simulink model "practica2"  (Simulink 7.3)
settings: Solver=ode45  StartTime=0.0  StopTime=1000  RelTol=1e-3
undefined symbols (not defined in the file or in its folder): p
libraries: simeventsrouting1 x8, simeventssink1 x6, simeventsgenerators1 x4, simeventsattributes2 x4, simeventstiming1 x4, simeventsqueue1 x2, simeventsgates1 x2, simeventsserver1 x2
settings Model: Creator=Mario  LastModifiedBy=usuario
settings SimEventsCC: propDiagAttribOutput=1  propDiagFcnCallOutput=1  propDiagStatOutput=0

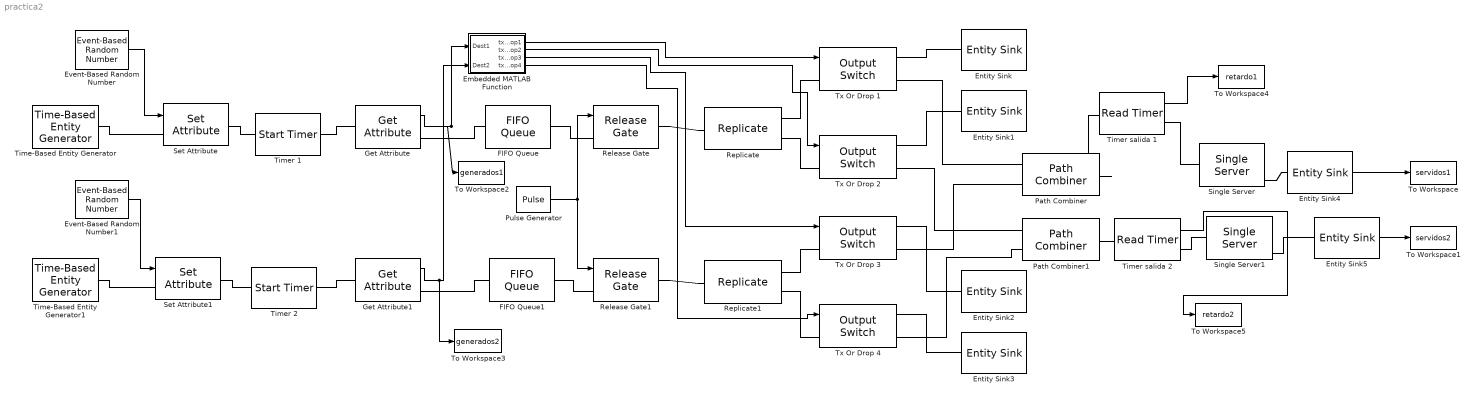
== system practica2 ==
  Embedded MATLAB Function : Stateflow chart
  Entity Sink{,1..3} (4 alike) : simeventssink1/Entity Sink  Priority=1  SystemSampleTime=-1  AvailableForArrivals=on  StatNumberArrived=Off
  Entity Sink4 : simeventssink1/Entity Sink  Priority=1  SystemSampleTime=-1  AvailableForArrivals=on  StatNumberArrived=On
  Entity Sink5 : simeventssink1/Entity Sink  Priority=1  SystemSampleTime=-1  AvailableForArrivals=on  StatNumberArrived=On
  Event-Based Random Number : simeventsgenerators1/Signal Generators/Event-Based Random Number  SystemSampleTime=-1  distribution=Arbitrary discrete  meanExp=1  minUnif=1  maxUnif=1  pOneBern=0.25  pSuccessBino=0.5  numTrialBino=1  meanNorm=0  stdNorm=1  minTri=1  maxTri=3  modeTri=2  thresholdLogn=0  scaleLogn=1  shapeLogn=1  pSuccessGeo=0.5  meanPoiss=1  thresholdLogl=0  scaleLogl=1  thresholdGam=0  scaleGam=1  shapeGam=1  minBeta=0  maxBeta=1  shape1Beta=1  shape2Beta=1  minUnid=0  maxUnid=1  numValueUnid=2  thresholdWbl=0  scaleWbl=1  shapeWbl=1  valueVecCont=[0 1]  cdfVecCont=[0 1]  valueVecDisc=[0 1 2]  probVecDisc=[1-p p/2 p/2]  seed=12345  IsProcessed=on  isConnected=1
  Event-Based Random Number1 : simeventsgenerators1/Signal Generators/Event-Based Random Number  SystemSampleTime=-1  distribution=Arbitrary discrete  meanExp=1  minUnif=1  maxUnif=1  pOneBern=0.25  pSuccessBino=0.5  numTrialBino=1  meanNorm=0  stdNorm=1  minTri=1  maxTri=3  modeTri=2  thresholdLogn=0  scaleLogn=1  shapeLogn=1  pSuccessGeo=0.5  meanPoiss=1  thresholdLogl=0  scaleLogl=1  thresholdGam=0  scaleGam=1  shapeGam=1  minBeta=0  maxBeta=1  shape1Beta=1  shape2Beta=1  minUnid=0  maxUnid=1  numValueUnid=2  thresholdWbl=0  scaleWbl=1  shapeWbl=1  valueVecCont=[0 1]  cdfVecCont=[0 1]  valueVecDisc=[0 1 2]  probVecDisc=[1-p p/2 p/2]  seed=76543  IsProcessed=on  isConnected=1
  FIFO Queue : simeventsqueue1/FIFO Queue  Priority=1  SystemSampleTime=-1  Capacity=1  EnableTOPort=off  StatNumberDeparted=Off  StatNumberInBlock=Off  StatPendingEntity=Off  StatAverageWait=Off  StatAverageQueueLength=Off  StatNumberTimedout=Off
  FIFO Queue1 : simeventsqueue1/FIFO Queue  Priority=1  SystemSampleTime=-1  Capacity=1  EnableTOPort=off  StatNumberDeparted=Off  StatNumberInBlock=Off  StatPendingEntity=Off  StatAverageWait=Off  StatAverageQueueLength=Off  StatNumberTimedout=Off
  Get Attribute : simeventsattributes2/Get Attribute  Priority=1  DialogController=des_ddg_create  DialogControllerArgs=DataTag9  SystemSampleTime=-1  AttributeName=Attribute1  AttributeMissing=Error  AttributeDefaultValue=1  AttributeSendTiming=After entity departure  AttributeTreatAsVector=1  StatNumberDeparted=Off  EvaluatedDefaultAttributeValue={[]}
  Get Attribute1 : simeventsattributes2/Get Attribute  Priority=1  DialogController=des_ddg_create  DialogControllerArgs=DataTag11  SystemSampleTime=-1  AttributeName=Attribute1  AttributeMissing=Error  AttributeDefaultValue=1  AttributeSendTiming=After entity departure  AttributeTreatAsVector=1  StatNumberDeparted=Off  EvaluatedDefaultAttributeValue={[]}
  Path Combiner : simeventsrouting1/Path Combiner  Priority=1  SystemSampleTime=-1  NumberInputPorts=2  InputPortPrecedence=IN1 port  InitialSeed=45675  SpecifyEventPriority=off  PriorityPathCombinerPortPrecedenceSelection=4100  StatNumberDeparted=Off  StatLastArrivalPort=Off  EvaluatedNumPorts=2
  Path Combiner1 : simeventsrouting1/Path Combiner  Priority=1  SystemSampleTime=-1  NumberInputPorts=2  InputPortPrecedence=IN1 port  InitialSeed=45675  SpecifyEventPriority=off  PriorityPathCombinerPortPrecedenceSelection=4100  StatNumberDeparted=Off  StatLastArrivalPort=Off  EvaluatedNumPorts=2
  Pulse Generator : DiscretePulseGenerator  Amplitude=1  Period=10  PulseWidth=5  PhaseDelay=3  SampleTime=0.1
  Release Gate : simeventsgates1/Release Gate  Priority=1  SystemSampleTime=-1  OpenGateUpon=Change in signal from port vc  SignalEdgeOption=Rising  SpecifyEventPriority=off  PriorityGateRelease=2200  StatNumberDeparted=Off
  Release Gate1 : simeventsgates1/Release Gate  Priority=1  SystemSampleTime=-1  OpenGateUpon=Change in signal from port vc  SignalEdgeOption=Rising  SpecifyEventPriority=off  PriorityGateRelease=2200  StatNumberDeparted=Off
  Replicate : simeventsrouting1/Replicate  Priority=1  SystemSampleTime=-1  NumberOutputPorts=2  ReplicateEntityWhen=All entity output ports are not blocked  OutputPortPrecedence=OUT1 port  InitialSeed=56789  ActionUponBlocking=Discard entity  StatNumberArrived=Off  StatNumberDeparted=Off  EvaluatedNumPorts=2
  Replicate1 : simeventsrouting1/Replicate  Priority=1  SystemSampleTime=-1  NumberOutputPorts=2  ReplicateEntityWhen=All entity output ports are not blocked  OutputPortPrecedence=OUT1 port  InitialSeed=56789  ActionUponBlocking=Discard entity  StatNumberArrived=Off  StatNumberDeparted=Off  EvaluatedNumPorts=2
  Set Attribute : simeventsattributes2/Set Attribute  Priority=1  DialogController=des_ddg_create  DialogControllerArgs=DataTag19  SystemSampleTime=-1  AttributeFrom=Signal port  AttributeName=Attribute1  AttributeTreatAsVector=1  AttributeValue=1  AttributeCreate=on  StatNumberDeparted=Off  EvaluatedAttributeValue={[]}
  Set Attribute1 : simeventsattributes2/Set Attribute  Priority=1  DialogController=des_ddg_create  DialogControllerArgs=DataTag21  SystemSampleTime=-1  AttributeFrom=Signal port  AttributeName=Attribute1  AttributeTreatAsVector=1  AttributeValue=1  AttributeCreate=on  StatNumberDeparted=Off  EvaluatedAttributeValue={[]}
  Single Server : simeventsserver1/Single Server  Priority=1  SystemSampleTime=-1  ServiceTimeFrom=Dialog  ServiceTime=0.99999  AttributeName=ServiceTime  PriorityServiceCompletion=500  PermitPreemption=off  SortingAttributeName=PriorityAttributeName  SortingDirection=Ascending  WriteToAttribute=off  ResidualAttributeName=ResidualServiceTime  CreateAttribute=on  EnableTOPort=off  StatNumberDeparted=On  StatNumberInBlock=Off  StatNumberPreempted=Off  StatPendingEntity=Off  StatAverageWait=Off  StatUtilization=On  StatNumberTimedout=Off
  Single Server1 : simeventsserver1/Single Server  Priority=1  SystemSampleTime=-1  ServiceTimeFrom=Dialog  ServiceTime=0.99999  AttributeName=ServiceTime  PriorityServiceCompletion=500  PermitPreemption=off  SortingAttributeName=PriorityAttributeName  SortingDirection=Ascending  WriteToAttribute=off  ResidualAttributeName=ResidualServiceTime  CreateAttribute=on  EnableTOPort=off  StatNumberDeparted=On  StatNumberInBlock=Off  StatNumberPreempted=Off  StatPendingEntity=Off  StatAverageWait=Off  StatUtilization=On  StatNumberTimedout=Off
  Time-Based Entity Generator : simeventsgenerators1/Entity Generators/Time-Based Entity Generator  Priority=1  DialogController=des_ddg_create  DialogControllerArgs=DataTag25  SystemSampleTime=-1  GenerateEntitiesUpon=Intergeneration time from dialog  Distribution=Constant  Minimum=0  Maximum=1  Mean=1  InitialSeed=12345  Period=1  PriorityEntityGeneration=300  GenerateEntityAtSimulationStart=on  ResponseWhenBlocked=Pause generation  ResponseWhenUnblocked=Immediate restart  EntityType=Blank  StatNumberDeparted=Off  StatPendingEntity=Off  StatAverageIntergenerationTime=Off
  Time-Based Entity Generator1 : simeventsgenerators1/Entity Generators/Time-Based Entity Generator  Priority=1  DialogController=des_ddg_create  DialogControllerArgs=DataTag27  SystemSampleTime=-1  GenerateEntitiesUpon=Intergeneration time from dialog  Distribution=Constant  Minimum=0  Maximum=1  Mean=1  InitialSeed=12345  Period=1  PriorityEntityGeneration=300  GenerateEntityAtSimulationStart=on  ResponseWhenBlocked=Pause generation  ResponseWhenUnblocked=Immediate restart  EntityType=Blank  StatNumberDeparted=Off  StatPendingEntity=Off  StatAverageIntergenerationTime=Off
  Timer 1 : simeventstiming1/Start Timer  Priority=0  SystemSampleTime=-1  TimerTag=T1  TimerStartedOption=Warn and continue  StatNumberDeparted=Off
  Timer 2 : simeventstiming1/Start Timer  Priority=0  SystemSampleTime=-1  TimerTag=T1  TimerStartedOption=Warn and continue  StatNumberDeparted=Off
  Timer salida 1 : simeventstiming1/Read Timer  Priority=0  SystemSampleTime=-1  TimerTag=T1  TimerModeOption=Error  TimerStop=off  StatNumberDeparted=Off  StatTimerNumberDeparted=Off  StatTimeElapsed=On  StatAverageTimeElapsed=Off
  Timer salida 2 : simeventstiming1/Read Timer  Priority=0  SystemSampleTime=-1  TimerTag=T1  TimerModeOption=Error  TimerStop=off  StatNumberDeparted=Off  StatTimerNumberDeparted=Off  StatTimeElapsed=On  StatAverageTimeElapsed=Off
  To Workspace : ToWorkspace  VariableName=servidos1  SampleTime=-1  SaveFormat=Array
  To Workspace1 : ToWorkspace  VariableName=servidos2  SampleTime=-1  SaveFormat=Array
  To Workspace2 : ToWorkspace  VariableName=generados1  SampleTime=1  SaveFormat=Array
  To Workspace3 : ToWorkspace  VariableName=generados2  SampleTime=1  SaveFormat=Array
  To Workspace4 : ToWorkspace  VariableName=retardo1  SampleTime=-1  SaveFormat=Array
  To Workspace5 : ToWorkspace  VariableName=retardo2  SampleTime=-1  SaveFormat=Array
  Tx Or Drop {1..4} (4 alike) : simeventsrouting1/Output Switch  Priority=1  SystemSampleTime=-1  NumberOutputPorts=2  SwitchingCriterion=From signal port p  InitialSeed=34567  AttributeName=Attribute1  InitialConditionsOpt=off  InitialConditions=1  EntityBufferOpt=off  SpecifyEventPriority=off  PriorityOutputSwitchSelectPort=4100  TimeoutPortOpt=off  StatNumberDeparted=Off  StatNumberTimedOut=Off  StatPendingEntity=Off  StatLastDeparturePort=Off  EvaluatedNumPorts=2
  wires:
  Event-Based Random Number/1 -> Set Attribute/1
  Event-Based Random Number1/1 -> Set Attribute1/1
  Get Attribute1/1 -> Embedded MATLAB Function/2(Dest2), To Workspace3/1
  Get Attribute/1 -> Embedded MATLAB Function/1(Dest1), To Workspace2/1
  Pulse Generator/1 -> Release Gate/1, Release Gate1/1
  Embedded MATLAB Function/1(tx_drop1) -> Tx Or Drop 1/1
  Embedded MATLAB Function/2(tx_drop2) -> Tx Or Drop 2/1
  Embedded MATLAB Function/3(tx_drop3) -> Tx Or Drop 3/1
  Embedded MATLAB Function/4(tx_drop4) -> Tx Or Drop 4/1
  Entity Sink4/1 -> To Workspace/1
  Entity Sink5/1 -> To Workspace1/1
  Timer salida 2/1 -> To Workspace5/1
  Timer salida 1/1 -> To Workspace4/1
  connections:
  Time-Based Entity Generator/RConn1 -- Set Attribute/LConn1
  Time-Based Entity Generator1/RConn1 -- Set Attribute1/LConn1
  Get Attribute1/RConn1 -- FIFO Queue1/LConn1
  FIFO Queue/RConn1 -- Release Gate/LConn1
  FIFO Queue1/RConn1 -- Release Gate1/LConn1
  Release Gate/RConn1 -- Replicate/LConn1
  Release Gate1/RConn1 -- Replicate1/LConn1
  Replicate/RConn1 -- Tx Or Drop 1/LConn1
  Replicate/RConn2 -- Tx Or Drop 2/LConn1
  Replicate1/RConn1 -- Tx Or Drop 3/LConn1
  Replicate1/RConn2 -- Tx Or Drop 4/LConn1
  Tx Or Drop 3/RConn1 -- Entity Sink2/LConn1
  Tx Or Drop 4/RConn1 -- Entity Sink3/LConn1
  Tx Or Drop 1/RConn1 -- Entity Sink/LConn1
  Tx Or Drop 2/RConn1 -- Entity Sink1/LConn1
  Tx Or Drop 1/RConn2 -- Path Combiner/LConn1
  Tx Or Drop 2/RConn2 -- Path Combiner1/LConn1
  Tx Or Drop 3/RConn2 -- Path Combiner/LConn2
  Tx Or Drop 4/RConn2 -- Path Combiner1/LConn2
  Get Attribute/RConn1 -- FIFO Queue/LConn1
  Set Attribute/RConn1 -- Timer 1/LConn1
  Timer 1/RConn1 -- Get Attribute/LConn1
  Set Attribute1/RConn1 -- Timer 2/LConn1
  Timer 2/RConn1 -- Get Attribute1/LConn1
  Single Server1/RConn1 -- Entity Sink5/LConn1
  Timer salida 2/RConn1 -- Single Server1/LConn1
  Path Combiner1/RConn1 -- Timer salida 2/LConn1
  Single Server/RConn1 -- Entity Sink4/LConn1
  Path Combiner/RConn1 -- Timer salida 1/LConn1
  Timer salida 1/RConn1 -- Single Server/LConn1

== matlab function Embedded MATLAB Function ==
  data: Dest1 input double; Dest2 input double; tx_drop1 output double; tx_drop2 output double; tx_drop3 output double; tx_drop4 output double
function [tx_drop1, tx_drop2, tx_drop3, tx_drop4] = port_selection_line1(Dest1, Dest2)

MatrizPuntosCruce = ones(2,2);

% Se cierran los puntos de cruce en la Matriz de Barras Cruzadas

if (Dest1 ~= 0)                     %Si la celda en la línea 1 no está vacía
    MatrizPuntosCruce(1,Dest1) = 2; % Se cierra el punto de cruce en
                                    % la primera fila
end

if (Dest2 ~= 0)                    %Si la celda en la línea 2 no está vacía
    MatrizPuntosCruce(2,Dest2) = 2;% Se cierra el punto de cruce en
                                   % la segunda fila
end

% Si hay contención en el puerto de salida 1

if (MatrizPuntosCruce(1,1)==2) && (MatrizPuntosCruce(2,1)==2)
    MatrizPuntosCruce(round(rand)+1,1)=1;
end

% Si hay contención en el puerto de salida 2

if (MatrizPuntosCruce(1,2)==2) && (MatrizPuntosCruce(2,2)==2)
    MatrizPuntosCruce(round(rand)+1,2)=1;
end

tx_drop1 = MatrizPuntosCruce(1,1);
tx_drop2 = MatrizPuntosCruce(1,2);
tx_drop3 = MatrizPuntosCruce(2,1);
tx_drop4 = MatrizPuntosCruce(2,2);
